simulink library "ddm"  (R2021b)
settings: Solver=VariableStepAuto  StartTime=0.0  StopTime=10.0  RelTol=1e-3
undefined symbols (not defined in the file or in its folder): ENUM_ADASACCSTA_ERROR, ENUM_ADASACCSTA_OFF, ENUM_ADASACCSTA_STANDBY, ENUM_ADASISASTA_OFF, ENUM_ALLOWMOV_ALLOWREADY, ENUM_APS, ENUM_BRKSTA_ERROR, ENUM_BRKSTA_OFF, ENUM_BRKSTA_ON, ENUM_CHGPREACTERRSTA_OBCPRE, ENUM_DCDCFAULTSTA_ANYFAULTLV1, ENUM_DCDCFAULTSTA_ANYFAULTLV2, ENUM_DRIVETRAIN_AWD, ENUM_DRIVETRAIN_FWD, ENUM_DRIVETRAIN_RWD, ENUM_DRSEATSTA_INVALID, ENUM_EDUDRTSTA_NORMAL, ENUM_EPBSTA_APPLIED, ENUM_EPBSTA_RELEASED, ENUM_HVBATTREADYPRE_READY, ENUM_MCUWARN_LV0, ENUM_MCUWARN_LV1, ENUM_MCUWARN_LV2, ENUM_MCUWARN_LV3, ENUM_MCUWARN_NOERROR, ENUM_OBCFAULTSTA_ANYFAULT, ENUM_PAS_R2F2, ENUM_PDFAULT_BATTPDFAIL, ENUM_PDFAULT_DCDCDISABLE, ENUM_PDFAULT_MCUDISABLE, ENUM_PDFAULT_MCUDISCHRG, ENUM_POWERSTA_OFF, ENUM_POWERSTA_ON, ENUM_POWERSTA_READY, ENUM_POWERSTA_STANDBY, ENUM_PRESSINDI_LOW, ENUM_PUFAULT_BATTUPFAIL, ENUM_PUFAULT_DCDCENABLEFAIL, ENUM_PUFAULT_PRECHRGCHKFAIL, ENUM_PUFAULT_SAFETYCHKFAIL, ENUM_PUSTATE_COMPLETED, ENUM_PWRSTASW_OFF, ENUM_PWRSTASW_OFFA, ENUM_PWRSTASW_OFFCHVCHRG, ENUM_PWRSTASW_OFFCLVCHRG, ENUM_PWRSTASW_ON, ENUM_PWRSTASW_ONHVCHRG, ENUM_PWRSTASW_READY, ENUM_PWRSTASW_STANDBY, ENUM_RANGESTA_12IN, ENUM_RANGESTA_12OUT, ENUM_SHIFTCOMMAND_D, ENUM_SHIFTCOMMAND_N, ENUM_SHIFTCOMMAND_P, ENUM_SHIFTCOMMAND_R, ENUM_ZONEMALFUNLV_1ST, ENUM_ZONEMALFUNLV_2ND, ENUM_ZONEMALFUNLV_3RD, ENUM_ZONEMALFUNLV_4TH, ENUM_ZONESPDCTRLMODE_ACC ... (+832)
libraries: hcu_lib x738, $bdroot x26, simulink x7
(part 10 of 25)

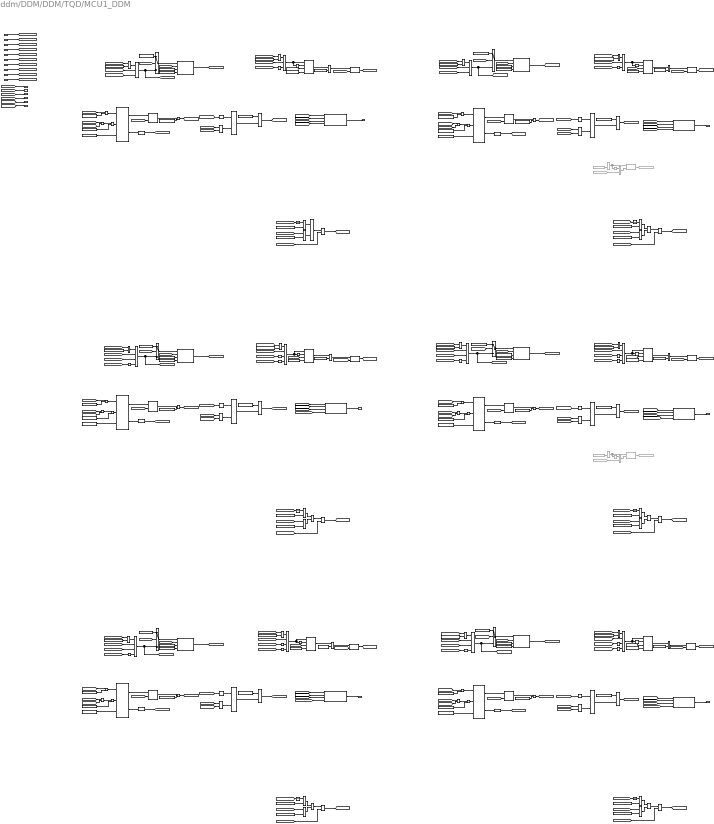
== system ddm/DDM/DDM/TQD/MCU1_DDM ==
  note: MCU_F1 Lost Comm (MCUF1NoCom)
  note: MCU_R1 Lost Comm (MCUR1NoCom)
  note: MCU_R1 Rolling Count Error (MCUR1RCErr)
  note: MCU_F1 Rolling Count Error (MCUF1RCErr)
  note: MCU_R1 Checksum Error (MCUR1CSErr)
  note: MCU_F1 Checksum Error (MCUF1CSErr)
  task_time_s : Inport
  VPMM_SysPwrSta_enum : Inport  Port=2
  No_CAN3_BUS_OFF : Inport  Port=3
  VDDM_MCUF1NoCom_flg : Inport  Port=4
  VDDM_MCUR1NoCom_flg : Inport  Port=5
  VDDM_MCUF1RCErr_flg : Inport  Port=6
  VDDM_MCUF1CSErr_flg : Inport  Port=7
  VDDM_MCUR1RCErr_flg : Inport  Port=8
  VDDM_MCUR1CSErr_flg : Inport  Port=9
  DTC_clear_request : Inport  Port=10
  Constant{1..2,9,24,35,46,53..54,62,66,79,86} (12 alike) : Constant  Value=ENUM_PWRSTASW_OFF
  Constant{3,10,25,40,55,75} (6 alike) : Constant  Value=ENUM_POWERSTA_OFF
  Constant{4,11,26,42,56,76} (6 alike) : Constant  Value=ENUM_POWERSTA_STANDBY
  Constant12 : Constant  Value=KDDM_MCUF1NoComDetSW_flg
  Constant13 : Constant  Value=KDDM_MCUF1NoComPassSW_flg
  Constant14 : Constant  Value=KDDM_MCUF1NoComDTC_cnt
  Constant15 : Constant  Value=KDDM_MCUF1NoComDFSSW_flg
  Constant16 : Constant  Value=KDDM_MCUR1NoComDTC_cnt
  Constant17 : Constant  Value=KDDM_MCUR1NoComPassTO_s
  Constant18 : Constant  Value=KDDM_MCUR1NoComPassTO_s
  Constant19 : Constant  Value=KDDM_MCUR1NoComDetTO_s
  Constant20 : Constant  Value=KDDM_MCUF1NoComCFSSW_flg
  Constant21 : Constant  Value=KDDM_MCUR1NoComCFSSW_flg
  Constant{22..23,38..39,73..74} (6 alike) : Constant  Value=FALSE
  Constant27 : Constant  Value=KDDM_MCUF1RCErrDetSW_flg
  Constant28 : Constant  Value=KDDM_MCUF1RCErrPassSW_flg
  Constant29 : Constant  Value=KDDM_MCUF1RCErrDTC_cnt
  Constant30 : Constant  Value=KDDM_MCUF1RCErrDFSSW_flg
  Constant31 : Constant  Value=KDDM_MCUR1RCErrDTC_cnt
  Constant32 : Constant  Value=KDDM_MCUR1RCErrPassTO_s
  Constant33 : Constant  Value=KDDM_MCUR1RCErrPassTO_s
  Constant34 : Constant  Value=KDDM_MCUR1RCErrDetTO_s
  Constant36 : Constant  Value=KDDM_MCUF1RCErrCFSSW_flg
  Constant37 : Constant  Value=KDDM_MCUR1RCErrCFSSW_flg
  Constant41 : Constant  Commented=on  Value=KDDM_MCUR1RCErrPassTO_s
  Constant43 : Constant  Commented=on  Value=KDDM_MCUR1RCErrPassTO_s
  Constant44 : Constant  Value=KDDM_MCUR1RCErrDetSW_flg
  Constant45 : Constant  Value=KDDM_MCUR1RCErrPassSW_flg
  Constant47 : Constant  Value=KDDM_MCUF1RCErrDTC_cnt
  Constant48 : Constant  Value=KDDM_MCUF1RCErrPassTO_s
  Constant49 : Constant  Value=KDDM_MCUR1RCErrDTC_cnt
  Constant5 : Constant  Value=KDDM_MCUR1NoComDetSW_flg
  Constant50 : Constant  Value=KDDM_MCUF1RCErrPassTO_s
  Constant51 : Constant  Value=KDDM_MCUF1RCErrDetTO_s
  Constant52 : Constant  Value=KDDM_MCUR1RCErrDFSSW_flg
  Constant57 : Constant  Value=KDDM_MCUF1CSErrDetSW_flg
  Constant58 : Constant  Value=KDDM_MCUF1CSErrPassSW_flg
  Constant59 : Constant  Value=KDDM_MCUF1CSErrDTC_cnt
  Constant6 : Constant  Value=KDDM_MCUR1NoComPassSW_flg
  Constant60 : Constant  Value=KDDM_MCUF1CSErrDFSSW_flg
  Constant61 : Constant  Value=KDDM_MCUR1CSErrDTC_cnt
  Constant63 : Constant  Value=KDDM_MCUR1CSErrPassTO_s
  Constant64 : Constant  Value=KDDM_MCUR1CSErrPassTO_s
  Constant65 : Constant  Value=KDDM_MCUR1CSErrDetTO_s
  Constant67 : Constant  Value=KDDM_MCUF1CSErrCFSSW_flg
  Constant68 : Constant  Value=KDDM_MCUF1NoComDTC_cnt
  Constant69 : Constant  Value=KDDM_MCUF1NoComPassTO_s
  Constant7 : Constant  Value=KDDM_MCUR1NoComDTC_cnt
  Constant70 : Constant  Value=KDDM_MCUF1NoComPassTO_s
  Constant71 : Constant  Value=KDDM_MCUF1NoComDetTO_s
  Constant72 : Constant  Value=KDDM_MCUR1CSErrCFSSW_flg
  Constant77 : Constant  Value=KDDM_MCUR1CSErrDetSW_flg
  Constant78 : Constant  Value=KDDM_MCUR1CSErrPassSW_flg
  Constant8 : Constant  Value=KDDM_MCUR1NoComDFSSW_flg
  Constant80 : Constant  Value=KDDM_MCUF1CSErrDTC_cnt
  Constant81 : Constant  Value=KDDM_MCUF1CSErrPassTO_s
  Constant82 : Constant  Value=KDDM_MCUR1CSErrDTC_cnt
  Constant83 : Constant  Value=KDDM_MCUF1CSErrPassTO_s
  Constant84 : Constant  Value=KDDM_MCUF1CSErrDetTO_s
  Constant85 : Constant  Value=KDDM_MCUR1CSErrDFSSW_flg
  DTC_Couter{1..6} (6 alike) : hcu_lib/Basic_Blocks/DTC_Couter
  DTC_Info{,1..5} (6 alike) : hcu_lib/Basic_Blocks/DTC_Info
  Data Type Conversion{1..6} (6 alike) : DataTypeConversion  OutDataTypeStr=uint8
  Equal{1..2,5,9..11,16,20..22,24,29} (12 alike) : RelationalOperator  Operator=~=  OutDataTypeStr=boolean  RndMeth=Simplest
  Equal12 : RelationalOperator  Commented=on  OutDataTypeStr=boolean  RndMeth=Simplest
  Equal{6,13,17,25,28,30} (6 alike) : RelationalOperator  OutDataTypeStr=boolean  RndMeth=Simplest
  Equal{3..4,7..8,14..15,18..19,26..27,31..32} (12 alike) : RelationalOperator  Operator===  OutDataTypeStr=boolean  RndMeth=Simplest
  Equal23 : RelationalOperator  Commented=on  OutDataTypeStr=boolean  RndMeth=Simplest
  From76 : From  Commented=on  GotoTag=VDDM_MCUR1RCErrRst_flg
  From94 : From  Commented=on  GotoTag=VDDM_MCUR1RCErrRst_flg
  Goto13 : Goto  Commented=on  GotoTag=VDDM_MCUR1RCErrPass_flg
  Goto14 : Goto  Commented=on  GotoTag=VDDM_MCUR1RCErrPass_flg
  Logical Operator{,1,4..7,10,16,18,25,27,36,38..42,49..50,55..57,60,63,69,71..75} (30 alike) : Logic  AllPortsSameDT=off  OutDataTypeStr=boolean
  Logical Operator{2,11,14,30} (4 alike) : Logic  Inputs=3  AllPortsSameDT=off  OutDataTypeStr=boolean
  Logical Operator{9,12,15,21,24,32,34,45..46,48,53,59,66,68,76..78,80} (18 alike) : Logic  Operator=OR  AllPortsSameDT=off  OutDataTypeStr=boolean
  Logical Operator{3,13,17,20,22,26,29,37,43,54,61,65,70,81..87} (20 alike) : Logic  Operator=NOT  AllPortsSameDT=off  OutDataTypeStr=boolean
  Logical Operator{19,23,28,31,51,58,64,67} (8 alike) : Logic  Inputs=4  AllPortsSameDT=off  OutDataTypeStr=boolean
  Logical Operator33 : Logic  Commented=on  Operator=NOT  AllPortsSameDT=off  OutDataTypeStr=boolean
  Logical Operator35 : Logic  Commented=on  Operator=NOT  AllPortsSameDT=off  OutDataTypeStr=boolean
  Logical Operator44 : Logic  Commented=on  Operator=OR  AllPortsSameDT=off  OutDataTypeStr=boolean
  Logical Operator62 : Logic  Commented=on  Operator=OR  AllPortsSameDT=off  OutDataTypeStr=boolean
  Relay{1..6} (6 alike) : Relay  OnSwitchValue=ONE_INT  OffSwitchValue=ZERO_INT
  SR_Latch{,1..4,6..9,11..19} (18 alike) : hcu_lib/Basic_Blocks/SR_Latch
  SR_Latch10 : hcu_lib/Basic_Blocks/SR_Latch  Commented=on
  SR_Latch5 : hcu_lib/Basic_Blocks/SR_Latch  Commented=on
  Switch{1..6} (6 alike) : Switch  Criteria=u2 ~= 0
  Test Detection Criteria{1..6} (6 alike) : hcu_lib/Basic_Blocks/Test Detection Criteria
  Timer{1..6} (6 alike) : hcu_lib/Basic_Blocks/Timer
  Unit Delay{,1..5} (6 alike) : UnitDelay  SampleTime=-1  HasFrameUpgradeWarning=on
  VDDM_MCUF1NoComDTC_raw32 : Outport
  VDDM_MCUR1NoComDTC_raw32 : Outport  Port=2
  VDDM_MCUF1RCErrDTC_raw32 : Outport  Port=3
  VDDM_MCUR1RCErrDTC_raw32 : Outport  Port=4
  VDDM_MCUF1CSErrDTC_raw32 : Outport  Port=5
  VDDM_MCUR1CSErrDTC_raw32 : Outport  Port=6
  VDDM_MCUF1NoComCFS_flg : Outport  Port=7
  VDDM_MCUF1RCErrCFS_flg : Outport  Port=8
  VDDM_MCUF1CSErrCFS_flg : Outport  Port=9
  VDDM_MCUR1NoComCFS_flg : Outport  Port=10
  VDDM_MCUR1RCErrCFS_flg : Outport  Port=11
  VDDM_MCUR1CSErrCFS_flg : Outport  Port=12
  wires:
  Constant12/1 -> Logical Operator5/2
  Equal3/1 -> Logical Operator4/1
  [VDDM_MCUF1NoCom_flg] -> Logical Operator30/3
  Constant10/1 -> Equal3/2
  Constant11/1 -> Equal4/2
  [DTC_clear_request] -> Logical Operator12/2
  Logical Operator12/1 -> [VDDM_MCUF1NoComCFSRls_flg]
  Equal21/1 -> Logical Operator30/1
  [VDDM_MCUF1NoComCFSRls_flg] -> SR_Latch/2
  Logical Operator5/1 -> DTC_Couter1/1
  Unit Delay/1 -> Equal3/1
  [No_CAN3_BUS_OFF] -> Logical Operator30/2
  Equal4/1 -> Logical Operator4/2
  [VPMM_SysPwrSta_enum] -> Unit Delay/1
  Timer1/1 -> Equal28/1
  DTC_Couter1/1 -> SR_Latch/1
  [VPMM_SysPwrSta_enum] -> Equal4/1
  [VDDM_MCUF1NoComDet_flg] -> Logical Operator5/1
  [VPMM_SysPwrSta_enum] -> Equal21/1
  Constant70/1 -> Timer1/4
  [task_time_s] -> Timer1/3
  Constant13/1 -> Logical Operator6/2
  Test Detection Criteria1/1 -> [VDDM_MCUF1NoComDet_flg]  "VDDM_MCUF1NoComDet_flg"
  Constant62/1 -> Equal21/2
  Logical Operator6/1 -> DTC_Couter1/2
  Logical Operator43/1 -> Timer1/2
  Constant69/1 -> Equal28/2
  Logical Operator4/1 -> Logical Operator12/1
  Logical Operator2/1 -> Logical Operator43/1, Timer1/1
  Equal1/1 -> Logical Operator2/1
  [VPMM_SysPwrSta_enum] -> Equal1/1
  [No_CAN3_BUS_OFF] -> Logical Operator2/2
  Constant1/1 -> Equal1/2
  [VDDM_MCUF1NoCom_flg] -> Logical Operator3/1
  Logical Operator3/1 -> Logical Operator2/3
  SR_Latch12/1 -> [VDDM_MCUF1NoComPass_flg]
  Logical Operator35/1 -> Logical Operator62/1
  Equal23/1 -> SR_Latch5/1, Logical Operator35/1
  From94/1 -> Logical Operator62/2
  Logical Operator62/1 -> SR_Latch5/2
  SR_Latch5/1 -> Goto14/1
  Constant41/1 -> Equal23/2
  [task_time_s] -> Test Detection Criteria1/2
  Constant68/1 -> Test Detection Criteria1/3
  Constant71/1 -> Test Detection Criteria1/4
  Equal28/1 -> SR_Latch12/1
  Constant14/1 -> DTC_Couter1/3
  [VDDM_MCUF1NoComPass_flg] -> Logical Operator34/1
  Logical Operator34/1 -> Logical Operator6/1
  [VDDM_MCUF1NoComCFSRls_flg] -> Logical Operator34/2
  Data Type Conversion2/1 -> [VDDM_MCUF1NoComDTC_cnt]  "VDDM_MCUF1NoComDTC_cnt"
  DTC_Couter1/2 -> Data Type Conversion2/1
  Constant15/1 -> Logical Operator55/1
  Logical Operator77/1 -> SR_Latch6/2
  Relay1/1 -> SR_Latch6/1
  Logical Operator55/1 -> [VDDM_MCUF1NoComDFS_flg]
  SR_Latch6/1 -> Logical Operator55/2
  [VDDM_MCUF1NoComDTC_cnt] -> Relay1/1
  [VDDM_MCUF1NoComDFSRls_flg] -> Logical Operator77/1
  [VDDM_MCUF1NoComCFS_flg] -> Logical Operator77/2
  Logical Operator66/1 -> SR_Latch13/2
  [VPMM_SysPwrSta_enum] -> Equal5/1
  [DTC_clear_request] -> Logical Operator9/2
  SR_Latch13/1 -> Logical Operator56/2
  Logical Operator17/1 -> Timer2/2
  [No_CAN3_BUS_OFF] -> Logical Operator11/2
  [VDDM_MCUR1NoComCFSRls_flg] -> SR_Latch1/2
  [VPMM_SysPwrSta_enum] -> Equal2/1
  Logical Operator16/1 -> Logical Operator9/1
  Equal5/1 -> Logical Operator14/1
  Relay2/1 -> SR_Latch13/1
  Constant19/1 -> Test Detection Criteria2/4
  Logical Operator57/1 -> DTC_Couter2/2
  Logical Operator11/1 -> Logical Operator17/1, Timer2/1
  Equal2/1 -> Logical Operator11/1
  [VDDM_MCUR1NoCom_flg] -> Logical Operator13/1
  Timer2/1 -> Equal6/1
  Equal7/1 -> Logical Operator16/1
  SR_Latch2/1 -> [VDDM_MCUR1NoComPass_flg]
  DTC_Couter2/2 -> Data Type Conversion1/1
  Constant3/1 -> Equal7/2
  [VDDM_MCUR1NoComDet_flg] -> Logical Operator18/1
  Constant5/1 -> Logical Operator18/2
  Test Detection Criteria2/1 -> [VDDM_MCUR1NoComDet_flg]  "VDDM_MCUR1NoComDet_flg"
  Logical Operator18/1 -> DTC_Couter2/1
  [VDDM_MCUR1NoComCFSRls_flg] -> Logical Operator15/2
  [VDDM_MCUR1NoComDFSRls_flg] -> Logical Operator66/1
  [VDDM_MCUR1NoComPass_flg] -> Logical Operator15/1
  [VDDM_MCUR1NoComDTC_cnt] -> Relay2/1
  Constant16/1 -> Test Detection Criteria2/3
  [VDDM_MCUR1NoComCFS_flg] -> Logical Operator66/2
  [VPMM_SysPwrSta_enum] -> Equal8/1
  Equal6/1 -> SR_Latch2/1
  [VDDM_MCUR1NoCom_flg] -> Logical Operator14/3
  Equal8/1 -> Logical Operator16/2
  Unit Delay1/1 -> Equal7/1
  Logical Operator15/1 -> Logical Operator57/1
  Constant2/1 -> Equal2/2
  Constant8/1 -> Logical Operator56/1
  Data Type Conversion1/1 -> [VDDM_MCUR1NoComDTC_cnt]  "VDDM_MCUR1NoComDTC_cnt"
  Logical Operator56/1 -> [VDDM_MCUR1NoComDFS_flg]
  Constant7/1 -> DTC_Couter2/3
  Constant4/1 -> Equal8/2
  Constant6/1 -> Logical Operator57/2
  Logical Operator9/1 -> [VDDM_MCUR1NoComCFSRls_flg]
  Constant18/1 -> Timer2/4
  Constant9/1 -> Equal5/2
  DTC_Couter2/1 -> SR_Latch1/1
  [No_CAN3_BUS_OFF] -> Logical Operator14/2
  [VPMM_SysPwrSta_enum] -> Unit Delay1/1
  Logical Operator13/1 -> Logical Operator11/3
  [task_time_s] -> Test Detection Criteria2/2
  Constant17/1 -> Equal6/2
  [task_time_s] -> Timer2/3
  [VDDM_MCUF1NoComCFS_flg] -> DTC_Info/3
  [VDDM_MCUF1NoComPass_flg] -> DTC_Info/2
  [VDDM_MCUF1NoComDet_flg] -> DTC_Info/1
  DTC_Info/1 -> VDDM_MCUF1NoComDTC_raw32/1  "VDDM_MCUF1NoComDTC_raw32"
  [VDDM_MCUR1NoComDet_flg] -> DTC_Info1/1
  DTC_Info1/1 -> VDDM_MCUR1NoComDTC_raw32/1  "VDDM_MCUR1NoComDTC_raw32"
  [VDDM_MCUR1NoComCFS_flg] -> DTC_Info1/3
  [VDDM_MCUR1NoComPass_flg] -> DTC_Info1/2
  task_time_s/1 -> [task_time_s]
  VPMM_SysPwrSta_enum/1 -> [VPMM_SysPwrSta_enum]
  No_CAN3_BUS_OFF/1 -> [No_CAN3_BUS_OFF]
  VDDM_MCUF1NoCom_flg/1 -> [VDDM_MCUF1NoCom_flg]
  DTC_clear_request/1 -> [DTC_clear_request]
  VDDM_MCUR1NoCom_flg/1 -> [VDDM_MCUR1NoCom_flg]
  SR_Latch/1 -> Logical Operator/1
  Logical Operator/1 -> [VDDM_MCUF1NoComCFS_flg]
  Constant20/1 -> Logical Operator/2
  Constant21/1 -> Logical Operator1/2
  SR_Latch1/1 -> Logical Operator1/1
  Logical Operator1/1 -> [VDDM_MCUR1NoComCFS_flg]
  [DTC_clear_request] -> DTC_Info/4
  [DTC_clear_request] -> DTC_Info1/4
  [DTC_clear_request] -> Switch6/2
  Switch6/1 -> Test Detection Criteria1/1
  Constant22/1 -> Switch6/1
  Logical Operator30/1 -> [VDDM_MCUF1NoComRst_flg], Switch6/3
  [DTC_clear_request] -> Switch1/2
  Switch1/1 -> Test Detection Criteria2/1
  Constant23/1 -> Switch1/1
  Equal14/1 -> Logical Operator36/1
  Unit Delay2/1 -> Equal14/1
  [VPMM_SysPwrSta_enum] -> Unit Delay2/1
  [VPMM_SysPwrSta_enum] -> Equal11/1
  Logical Operator42/1 -> DTC_Couter3/2
  Constant26/1 -> Equal15/2
  Equal13/1 -> SR_Latch7/1
  [VDDM_MCUR1RCErrCFSRls_flg] -> SR_Latch4/2
  [No_CAN3_BUS_OFF] -> Logical Operator31/2
  [VDDM_MCUF1RCErrCFSRls_flg] -> SR_Latch3/2
  Logical Operator37/1 -> Timer3/2
  [VDDM_MCUF1RCErrCFS_flg] -> Logical Operator46/2
  [DTC_clear_request] -> Logical Operator21/2
  [VPMM_SysPwrSta_enum] -> Equal15/1
  [VPMM_SysPwrSta_enum] -> Equal16/1
  Constant43/1 -> Equal12/2
  Timer3/1 -> Equal13/1
  Constant48/1 -> Equal13/2
  Logical Operator41/1 -> DTC_Couter4/2
  [VDDM_MCUR1RCErr_flg] -> Logical Operator22/1
  Equal15/1 -> Logical Operator36/2
  Logical Operator19/1 -> Timer4/1, Logical Operator26/1
  Test Detection Criteria3/1 -> [VDDM_MCUF1RCErrDet_flg]  "VDDM_MCUF1RCErrDet_flg"
  [VDDM_MCUF1RCErrCFSRls_flg] -> Logical Operator32/2
  Logical Operator44/1 -> SR_Latch10/2
  [VDDM_MCUF1RCErrDet_flg] -> Logical Operator38/1
  Constant51/1 -> Test Detection Criteria3/4
  [No_CAN3_BUS_OFF] -> Logical Operator28/2
  [VDDM_MCUR1RCErrDFSRls_flg] -> Logical Operator45/1
  Logical Operator32/1 -> Logical Operator42/1
  Constant30/1 -> Logical Operator39/1
  Equal11/1 -> Logical Operator31/1
  SR_Latch11/1 -> Logical Operator39/2
  [DTC_clear_request] -> Logical Operator48/2
  Logical Operator21/1 -> [VDDM_MCUF1RCErrCFSRls_flg]
  From76/1 -> Logical Operator44/2
  Data Type Conversion4/1 -> [VDDM_MCUF1RCErrDTC_cnt]  "VDDM_MCUF1RCErrDTC_cnt"
  Constant50/1 -> Timer3/4
  SR_Latch8/1 -> Logical Operator40/2
  [VPMM_SysPwrSta_enum] -> Equal9/1
  Constant34/1 -> Test Detection Criteria4/4
  [VDDM_MCUF1RCErr_flg] -> Logical Operator29/1
  [VDDM_MCUF1RCErrPass_flg] -> Logical Operator32/1
  [VDDM_MCUF1RCErrDFSRls_flg] -> Logical Operator46/1
  Constant46/1 -> Equal11/2
  Logical Operator46/1 -> SR_Latch11/2
  Constant29/1 -> DTC_Couter3/3
  Equal12/1 -> SR_Latch10/1, Logical Operator33/1
  SR_Latch9/1 -> [VDDM_MCUR1RCErrPass_flg]
  [VDDM_MCUF1RCErr_flg] -> Logical Operator31/3
  [VDDM_MCUR1RCErrCFSRls_flg] -> Logical Operator24/2
  [VPMM_SysPwrSta_enum] -> Equal10/1
  Relay4/1 -> SR_Latch8/1
  Equal10/1 -> Logical Operator19/1
  Logical Operator29/1 -> Logical Operator28/3
  Constant27/1 -> Logical Operator38/2
  Test Detection Criteria4/1 -> [VDDM_MCUR1RCErrDet_flg]  "VDDM_MCUR1RCErrDet_flg"
  [VDDM_MCUR1RCErrDet_flg] -> Logical Operator27/1
  Logical Operator36/1 -> Logical Operator21/1
  Relay3/1 -> SR_Latch11/1
  Constant25/1 -> Equal14/2
  SR_Latch10/1 -> Goto13/1
  Constant28/1 -> Logical Operator42/2
  DTC_Info2/1 -> VDDM_MCUF1RCErrDTC_raw32/1  "VDDM_MCUF1RCErrDTC_raw32"
  [VPMM_SysPwrSta_enum] -> Unit Delay3/1
  Constant35/1 -> Equal10/2
  DTC_Couter4/2 -> Data Type Conversion3/1
  Logical Operator33/1 -> Logical Operator44/1
  Constant42/1 -> Equal19/2
  [VDDM_MCUR1RCErrCFS_flg] -> Logical Operator45/2
  DTC_Couter4/1 -> SR_Latch4/1
  Constant40/1 -> Equal18/2
  DTC_Couter3/1 -> SR_Latch3/1
  Data Type Conversion3/1 -> [VDDM_MCUR1RCErrDTC_cnt]  "VDDM_MCUR1RCErrDTC_cnt"
  Constant52/1 -> Logical Operator40/1
  Logical Operator24/1 -> Logical Operator41/1
  Equal19/1 -> Logical Operator25/2
  [VDDM_MCUF1RCErrDet_flg] -> DTC_Info2/1
  Unit Delay3/1 -> Equal18/1
  [VDDM_MCUF1RCErrPass_flg] -> DTC_Info2/2
  DTC_Info3/1 -> VDDM_MCUR1RCErrDTC_raw32/1  "VDDM_MCUR1RCErrDTC_raw32"
  [task_time_s] -> Timer4/3
  [task_time_s] -> Test Detection Criteria3/2
  Constant24/1 -> Equal9/2
  [VDDM_MCUR1RCErrPass_flg] -> DTC_Info3/2
  Timer4/1 -> Equal17/1
  [VDDM_MCUR1RCErrPass_flg] -> Logical Operator24/1
  Logical Operator38/1 -> DTC_Couter3/1
  [VDDM_MCUR1RCErrDet_flg] -> DTC_Info3/1
  Logical Operator25/1 -> Logical Operator48/1
  Logical Operator27/1 -> DTC_Couter4/1
  Constant44/1 -> Logical Operator27/2
  [VDDM_MCUR1RCErr_flg] -> Logical Operator23/3
  Constant33/1 -> Timer4/4
  [No_CAN3_BUS_OFF] -> Logical Operator19/2
  Logical Operator40/1 -> [VDDM_MCUR1RCErrDFS_flg]
  [DTC_clear_request] -> Switch3/2
  Constant53/1 -> Equal16/2
  SR_Latch3/1 -> Logical Operator7/1
  [VDDM_MCUR1RCErrDTC_cnt] -> Relay4/1
  Logical Operator22/1 -> Logical Operator19/3
  Constant47/1 -> Test Detection Criteria3/3
  [task_time_s] -> Timer3/3
  Logical Operator39/1 -> [VDDM_MCUF1RCErrDFS_flg]
  Logical Operator7/1 -> [VDDM_MCUF1RCErrCFS_flg]
  SR_Latch7/1 -> [VDDM_MCUF1RCErrPass_flg]
  SR_Latch4/1 -> Logical Operator10/1
  Constant37/1 -> Logical Operator10/2
  Equal16/1 -> Logical Operator23/1
  [VDDM_MCUR1RCErrCFS_flg] -> DTC_Info3/3
  Logical Operator28/1 -> Timer3/1, Logical Operator37/1
  Constant32/1 -> Equal17/2
  [VDDM_MCUF1RCErrCFS_flg] -> DTC_Info2/3
  Constant45/1 -> Logical Operator41/2
  Logical Operator48/1 -> [VDDM_MCUR1RCErrCFSRls_flg]
  Constant38/1 -> Switch3/1
  Equal18/1 -> Logical Operator25/1
  [No_CAN3_BUS_OFF] -> Logical Operator23/2
  Equal17/1 -> SR_Latch9/1
  Constant49/1 -> DTC_Couter4/3
  Switch3/1 -> Test Detection Criteria3/1
  Logical Operator26/1 -> Timer4/2
  Constant31/1 -> Test Detection Criteria4/3
  Constant36/1 -> Logical Operator7/2
  [VPMM_SysPwrSta_enum] -> Equal19/1
  [DTC_clear_request] -> Switch2/2
  Logical Operator45/1 -> SR_Latch8/2
  [task_time_s] -> Test Detection Criteria4/2
  Switch2/1 -> Test Detection Criteria4/1
  Constant39/1 -> Switch2/1
  Logical Operator10/1 -> [VDDM_MCUR1RCErrCFS_flg]
  [DTC_clear_request] -> DTC_Info2/4
  [VDDM_MCUF1RCErrDTC_cnt] -> Relay3/1
  [DTC_clear_request] -> DTC_Info3/4
  DTC_Couter3/2 -> Data Type Conversion4/1
  Equal9/1 -> Logical Operator28/1
  Equal26/1 -> Logical Operator69/1
  Unit Delay4/1 -> Equal26/1
  [VPMM_SysPwrSta_enum] -> Unit Delay4/1
  [VPMM_SysPwrSta_enum] -> Equal24/1
  Logical Operator75/1 -> DTC_Couter5/2
  Constant56/1 -> Equal27/2
  Equal25/1 -> SR_Latch16/1
  [VDDM_MCUR1CSErrCFSRls_flg] -> SR_Latch15/2
  [No_CAN3_BUS_OFF] -> Logical Operator67/2
  [VDDM_MCUF1CSErrCFSRls_flg] -> SR_Latch14/2
  Logical Operator70/1 -> Timer5/2
  [VDDM_MCUF1CSErrCFS_flg] -> Logical Operator78/2
  [DTC_clear_request] -> Logical Operator53/2
  [VPMM_SysPwrSta_enum] -> Equal27/1
  [VPMM_SysPwrSta_enum] -> Equal29/1
  Timer5/1 -> Equal25/1
  Constant81/1 -> Equal25/2
  Logical Operator74/1 -> DTC_Couter6/2
  [VDDM_MCUR1CSErr_flg] -> Logical Operator54/1
  Equal27/1 -> Logical Operator69/2
  Logical Operator51/1 -> Timer6/1, Logical Operator61/1
  Test Detection Criteria5/1 -> [VDDM_MCUF1CSErrDet_flg]  "VDDM_MCUF1CSErrDet_flg"
  [VDDM_MCUF1CSErrCFSRls_flg] -> Logical Operator68/2
  [VDDM_MCUF1CSErrDet_flg] -> Logical Operator71/1
  Constant84/1 -> Test Detection Criteria5/4
  [No_CAN3_BUS_OFF] -> Logical Operator64/2
  [VDDM_MCUR1CSErrDFSRls_flg] -> Logical Operator76/1
  Logical Operator68/1 -> Logical Operator75/1
  Constant60/1 -> Logical Operator72/1
  Equal24/1 -> Logical Operator67/1
  SR_Latch19/1 -> Logical Operator72/2
  [DTC_clear_request] -> Logical Operator80/2
  Logical Operator53/1 -> [VDDM_MCUF1CSErrCFSRls_flg]
  Data Type Conversion6/1 -> [VDDM_MCUF1CSErrDTC_cnt]  "VDDM_MCUF1CSErrDTC_cnt"
  Constant83/1 -> Timer5/4
  SR_Latch17/1 -> Logical Operator73/2
  [VPMM_SysPwrSta_enum] -> Equal20/1
  Constant65/1 -> Test Detection Criteria6/4
  [VDDM_MCUF1CSErr_flg] -> Logical Operator65/1
  [VDDM_MCUF1CSErrPass_flg] -> Logical Operator68/1
  [VDDM_MCUF1CSErrDFSRls_flg] -> Logical Operator78/1
  Constant79/1 -> Equal24/2
  Logical Operator78/1 -> SR_Latch19/2
  Constant59/1 -> DTC_Couter5/3
  SR_Latch18/1 -> [VDDM_MCUR1CSErrPass_flg]
  [VDDM_MCUF1CSErr_flg] -> Logical Operator67/3
  [VDDM_MCUR1CSErrCFSRls_flg] -> Logical Operator59/2
  [VPMM_SysPwrSta_enum] -> Equal22/1
  Relay6/1 -> SR_Latch17/1
  Equal22/1 -> Logical Operator51/1
  Logical Operator65/1 -> Logical Operator64/3
  Constant57/1 -> Logical Operator71/2
  Test Detection Criteria6/1 -> [VDDM_MCUR1CSErrDet_flg]  "VDDM_MCUR1CSErrDet_flg"
  [VDDM_MCUR1CSErrDet_flg] -> Logical Operator63/1
  Logical Operator69/1 -> Logical Operator53/1
  Relay5/1 -> SR_Latch19/1
  Constant55/1 -> Equal26/2
  Constant58/1 -> Logical Operator75/2
  DTC_Info4/1 -> VDDM_MCUF1CSErrDTC_raw32/1  "VDDM_MCUF1CSErrDTC_raw32"
  [VPMM_SysPwrSta_enum] -> Unit Delay5/1
  Constant66/1 -> Equal22/2
  DTC_Couter6/2 -> Data Type Conversion5/1
  Constant76/1 -> Equal32/2
  [VDDM_MCUR1CSErrCFS_flg] -> Logical Operator76/2
  DTC_Couter6/1 -> SR_Latch15/1
  Constant75/1 -> Equal31/2
  DTC_Couter5/1 -> SR_Latch14/1
  Data Type Conversion5/1 -> [VDDM_MCUR1CSErrDTC_cnt]  "VDDM_MCUR1CSErrDTC_cnt"
  Constant85/1 -> Logical Operator73/1
  Logical Operator59/1 -> Logical Operator74/1
  Equal32/1 -> Logical Operator60/2
  [VDDM_MCUF1CSErrDet_flg] -> DTC_Info4/1
  Unit Delay5/1 -> Equal31/1
  [VDDM_MCUF1CSErrPass_flg] -> DTC_Info4/2
  DTC_Info5/1 -> VDDM_MCUR1CSErrDTC_raw32/1  "VDDM_MCUR1CSErrDTC_raw32"
  [task_time_s] -> Timer6/3
  [task_time_s] -> Test Detection Criteria5/2
  Constant54/1 -> Equal20/2
  [VDDM_MCUR1CSErrPass_flg] -> DTC_Info5/2
  Timer6/1 -> Equal30/1
  [VDDM_MCUR1CSErrPass_flg] -> Logical Operator59/1
  Logical Operator71/1 -> DTC_Couter5/1
  [VDDM_MCUR1CSErrDet_flg] -> DTC_Info5/1
  Logical Operator60/1 -> Logical Operator80/1
  Logical Operator63/1 -> DTC_Couter6/1
  Constant77/1 -> Logical Operator63/2
  [VDDM_MCUR1CSErr_flg] -> Logical Operator58/3
  Constant64/1 -> Timer6/4
  [No_CAN3_BUS_OFF] -> Logical Operator51/2
  Logical Operator73/1 -> [VDDM_MCUR1CSErrDFS_flg]
  [DTC_clear_request] -> Switch5/2
  Constant86/1 -> Equal29/2
  SR_Latch14/1 -> Logical Operator49/1
  [VDDM_MCUR1CSErrDTC_cnt] -> Relay6/1
  Logical Operator54/1 -> Logical Operator51/3
  Constant80/1 -> Test Detection Criteria5/3
  [task_time_s] -> Timer5/3
  Logical Operator72/1 -> [VDDM_MCUF1CSErrDFS_flg]
  Logical Operator49/1 -> [VDDM_MCUF1CSErrCFS_flg]
  SR_Latch16/1 -> [VDDM_MCUF1CSErrPass_flg]
  SR_Latch15/1 -> Logical Operator50/1
  Constant72/1 -> Logical Operator50/2
  Equal29/1 -> Logical Operator58/1
  [VDDM_MCUR1CSErrCFS_flg] -> DTC_Info5/3
  Logical Operator64/1 -> Timer5/1, Logical Operator70/1
  Constant63/1 -> Equal30/2
  [VDDM_MCUF1CSErrCFS_flg] -> DTC_Info4/3
  Constant78/1 -> Logical Operator74/2
  Logical Operator80/1 -> [VDDM_MCUR1CSErrCFSRls_flg]
  Constant73/1 -> Switch5/1
  Equal31/1 -> Logical Operator60/1
  [No_CAN3_BUS_OFF] -> Logical Operator58/2
  Equal30/1 -> SR_Latch18/1
  Constant82/1 -> DTC_Couter6/3
  Switch5/1 -> Test Detection Criteria5/1
  Logical Operator61/1 -> Timer6/2
  Constant61/1 -> Test Detection Criteria6/3
  Constant67/1 -> Logical Operator49/2
  [VPMM_SysPwrSta_enum] -> Equal32/1
  [DTC_clear_request] -> Switch4/2
  Logical Operator76/1 -> SR_Latch17/2
  [task_time_s] -> Test Detection Criteria6/2
  Switch4/1 -> Test Detection Criteria6/1
  Constant74/1 -> Switch4/1
  Logical Operator50/1 -> [VDDM_MCUR1CSErrCFS_flg]
  [DTC_clear_request] -> DTC_Info4/4
  [VDDM_MCUF1CSErrDTC_cnt] -> Relay5/1
  [DTC_clear_request] -> DTC_Info5/4
  DTC_Couter5/2 -> Data Type Conversion6/1
  Equal20/1 -> Logical Operator64/1
  [VDDM_MCUF1NoComCFS_flg] -> Logical Operator85/1
  [VDDM_MCUF1NoComCFS_flg] -> Logical Operator81/1
  Logical Operator81/1 -> Logical Operator31/4
  Logical Operator82/1 -> Logical Operator23/4
  [VDDM_MCUR1NoComCFS_flg] -> Logical Operator82/1
  Logical Operator83/1 -> Logical Operator67/4
  [VDDM_MCUF1NoComCFS_flg] -> Logical Operator83/1
  Logical Operator84/1 -> Logical Operator58/4
  [VDDM_MCUR1NoComCFS_flg] -> Logical Operator84/1
  VDDM_MCUF1RCErr_flg/1 -> [VDDM_MCUF1RCErr_flg]
  VDDM_MCUF1CSErr_flg/1 -> [VDDM_MCUF1CSErr_flg]
  VDDM_MCUR1RCErr_flg/1 -> [VDDM_MCUR1RCErr_flg]
  VDDM_MCUR1CSErr_flg/1 -> [VDDM_MCUR1CSErr_flg]
  Logical Operator85/1 -> Logical Operator28/4
  [VDDM_MCUF1NoComRst_flg] -> SR_Latch12/2
  [VDDM_MCUF1RCErrRst_flg] -> SR_Latch7/2
  Logical Operator31/1 -> [VDDM_MCUF1RCErrRst_flg], Switch3/3
  [VDDM_MCUR1NoComCFS_flg] -> Logical Operator20/1
  Logical Operator20/1 -> Logical Operator19/4
  Logical Operator86/1 -> Logical Operator51/4
  [VDDM_MCUR1NoComCFS_flg] -> Logical Operator86/1
  [VDDM_MCUF1NoComCFS_flg] -> Logical Operator87/1
  Logical Operator87/1 -> Logical Operator64/4
  Logical Operator67/1 -> [VDDM_MCUF1CSErrRst_flg], Switch5/3
  [VDDM_MCUF1CSErrRst_flg] -> SR_Latch16/2
  Logical Operator14/1 -> [VDDM_MCUR1NoComRst_flg], Switch1/3
  [VDDM_MCUR1NoComRst_flg] -> SR_Latch2/2
  Logical Operator23/1 -> [VDDM_MCUR1RCErrRst_flg], Switch2/3
  [VDDM_MCUR1RCErrRst_flg] -> SR_Latch9/2
  Logical Operator58/1 -> [VDDM_MCUR1CSErrRst_flg], Switch4/3
  [VDDM_MCUR1CSErrRst_flg] -> SR_Latch18/2
  [VDDM_MCUF1NoComCFS_flg] -> VDDM_MCUF1NoComCFS_flg/1
  [VDDM_MCUF1CSErrCFS_flg] -> VDDM_MCUF1CSErrCFS_flg/1
  [VDDM_MCUR1CSErrCFS_flg] -> VDDM_MCUR1CSErrCFS_flg/1
  [VDDM_MCUR1RCErrCFS_flg] -> VDDM_MCUR1RCErrCFS_flg/1
  [VDDM_MCUR1NoComCFS_flg] -> VDDM_MCUR1NoComCFS_flg/1
  [VDDM_MCUF1RCErrCFS_flg] -> VDDM_MCUF1RCErrCFS_flg/1

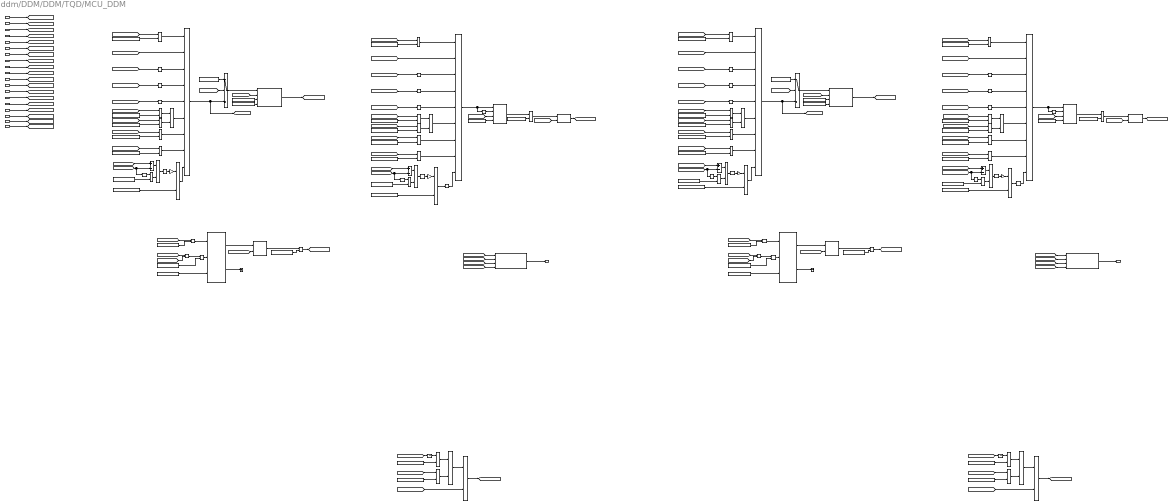
== system ddm/DDM/DDM/TQD/MCU_DDM ==
  note: Front Motor Torque Response Error (FrMCUTqErr)
  note: Fail Safe During Detection
  note: Test Pass Creteria
  note: Test Dtection Criteria
  note: Fail Safe After Detection
  note: Fail Safe During Detection
  note: Test Pass Creteria
  note: Rear Motor Torque Response Error (RrMCUTqErr)
  note: Test Dtection Criteria
  note: Fail Safe After Detection
  task_time_s : Inport
  VPMM_SysPwrSta_enum : Inport  Port=2
  No_CAN3_BUS_OFF : Inport  Port=3
  VDDM_MCUF1NoComCFS_flg : Inport  Port=4
  VDDM_MCUF1RCErrCFS_flg : Inport  Port=5
  VDDM_MCUF1CSErrCFS_flg : Inport  Port=6
  VINP_VehSpeed_kph : Inport  Port=7
  VINP_FrEDUDrtSta_flg : Inport  Port=8
  VINP_FrEDURealTMTq_Nm : Inport  Port=9
  VTQR_FrTMTqReq_Nm : Inport  Port=10
  VDDM_MCUR1NoComCFS_flg : Inport  Port=11
  VDDM_MCUR1RCErrCFS_flg : Inport  Port=12
  VDDM_MCUR1CSErrCFS_flg : Inport  Port=13
  VINP_RrEDUDrtSta_flg : Inport  Port=14
  VINP_RrEDURealTMTq_Nm : Inport  Port=15
  VTQR_RrTMTqReq_Nm : Inport  Port=16
  VINP_MCUWarnF_enum : Inport  Port=17
  VINP_MCUWarnR_enum : Inport  Port=18
  DTC_clear_request : Inport  Port=19
  Abs{,1..7} (8 alike) : Abs
  Add{,1..3} (4 alike) : Sum  Inputs=+-
  Constant{,1,47..48} (4 alike) : Constant  Value=eps
  Constant10 : Constant  Value=ENUM_POWERSTA_OFF
  Constant11 : Constant  Value=ENUM_POWERSTA_STANDBY
  Constant12 : Constant  Value=KDDM_RrMCUTqErrDetSW_flg
  Constant13 : Constant  Value=KDDM_FrMCUTqErrDetSW_flg
  Constant14 : Constant  Value=KDDM_FrMCUTqErrPassSW_flg
  Constant15 : Constant  Value=KDDM_FrMCUTqErrDet_pct
  Constant{4,16,26,32} (4 alike) : Constant  Value=ENUM_MCUWARN_LV0
  Constant{17,27,33,44} (4 alike) : Constant  Value=ENUM_PWRSTASW_OFF
  Constant18 : Constant  Value=ENUM_POWERSTA_OFF
  Constant19 : Constant  Value=ENUM_POWERSTA_STANDBY
  Constant2 : Constant  Value=KDDM_FrMCUTqErrCFSSW_flg
  Constant{5,20,29,34} (4 alike) : Constant  Value=ENUM_MCUWARN_NOERROR
  Constant{6,21,30,35} (4 alike) : Constant  Value=ENUM_EDUDRTSTA_NORMAL
  Constant22 : Constant  Value=KDDM_RrMCUTqErrPassSW_flg
  Constant23 : Constant  Value=KDDM_RrMCUTqErrCFSSW_flg
  Constant24 : Constant  Value=FALSE
  Constant25 : Constant  Value=KDDM_RrMCUTqErrDet_pct
  Constant28 : Constant  Value=KDDM_RrMCUTqErrDTC_cnt
  Constant3 : Constant  Value=KDDM_FrMCUTqErrDet_kph
  Constant31 : Constant  Value=KDDM_RrMCUTqErrDet_kph
  Constant36 : Constant  Value=KDDM_RrMCUTqErrPassTO_s
  Constant37 : Constant  Value=KDDM_RrMCUTqErrDetTO_s
  Constant38 : Constant  Value=KDDM_RrMCUTqErrDet_kph
  Constant39 : Constant  Value=KDDM_RrMCUTqErrPassTO_s
  Constant40 : Constant  Value=KDDM_RrMCUTqErrDTC_cnt
  Constant41 : Constant  Value=KDDM_FrMCUTqErrDet_pct
  Constant42 : Constant  Value=FALSE
  Constant43 : Constant  Value=KDDM_FrMCUTqErrDTC_cnt
  Constant45 : Constant  Value=KDDM_FrMCUTqErrPassTO_s
  Constant46 : Constant  Value=KDDM_FrMCUTqErrDetTO_s
  Constant7 : Constant  Value=KDDM_FrMCUTqErrDet_kph
  Constant70 : Constant  Value=KDDM_FrMCUTqErrPassTO_s
  Constant8 : Constant  Value=KDDM_FrMCUTqErrDTC_cnt
  Constant9 : Constant  Value=KDDM_RrMCUTqErrDet_pct
  DTC_Couter1 : hcu_lib/Basic_Blocks/DTC_Couter
  DTC_Couter2 : hcu_lib/Basic_Blocks/DTC_Couter
  DTC_Info : hcu_lib/Basic_Blocks/DTC_Info
  DTC_Info1 : hcu_lib/Basic_Blocks/DTC_Info
  Divide{,1..3} (4 alike) : Product  Inputs=*/
  Equal{1,3..4,6..10,15..16,21..22,30..31,33..34} (16 alike) : RelationalOperator  Operator===  OutDataTypeStr=boolean  RndMeth=Simplest
  Equal{5,11..12,17..18,27} (6 alike) : RelationalOperator  OutDataTypeStr=boolean  RndMeth=Simplest
  Equal{2,13,19,23} (4 alike) : RelationalOperator  Operator=>  OutDataTypeStr=boolean  RndMeth=Simplest
  Equal{14,20,24,26} (4 alike) : RelationalOperator  Operator=~=  OutDataTypeStr=boolean  RndMeth=Simplest
  Gain{,1..3} (4 alike) : Gain  Gain=100  OutDataTypeStr=single
  Logical Operator{1..2,5,12,16,20,25,31} (8 alike) : Logic  Operator=OR  AllPortsSameDT=off  OutDataTypeStr=boolean
  Logical Operator{3,7,9..10,13..15,17,21..23,26,28,34..35,37} (16 alike) : Logic  Operator=NOT  AllPortsSameDT=off  OutDataTypeStr=boolean
  Logical Operator{11,18,27,30} (4 alike) : Logic  Inputs=9  AllPortsSameDT=off  OutDataTypeStr=boolean
  Logical Operator{4,6,8,19,24,29,32..33} (8 alike) : Logic  AllPortsSameDT=off  OutDataTypeStr=boolean
  Max{,1..3} (4 alike) : MinMax  Function=max  Inputs=2
  SR_Latch{1..3,12} (4 alike) : hcu_lib/Basic_Blocks/SR_Latch
  Switch1 : Switch  Criteria=u2 ~= 0
  Switch6 : Switch  Criteria=u2 ~= 0
  Terminator : Terminator
  Terminator1 : Terminator
  Test Detection Criteria1 : hcu_lib/Basic_Blocks/Test Detection Criteria
  Test Detection Criteria2 : hcu_lib/Basic_Blocks/Test Detection Criteria
  Timer1 : hcu_lib/Basic_Blocks/Timer
  Timer2 : hcu_lib/Basic_Blocks/Timer
  Unit Delay : UnitDelay  SampleTime=-1  HasFrameUpgradeWarning=on
  Unit Delay1 : UnitDelay  SampleTime=-1  HasFrameUpgradeWarning=on
  VDDM_FrMCUTqErrDTC_raw32 : Outport
  VDDM_RrMCUTqErrDTC_raw32 : Outport  Port=2
  wires:
  Equal26/1 -> Logical Operator30/1
  Constant44/1 -> Equal26/2
  [VPMM_SysPwrSta_enum] -> Equal26/1
  Logical Operator12/1 -> [VDDM_FrMCUTqErrCFSRls_flg]
  Constant11/1 -> Equal4/2
  [VPMM_SysPwrSta_enum] -> Unit Delay/1
  [DTC_clear_request] -> Logical Operator12/2
  Equal3/1 -> Logical Operator4/1
  [VPMM_SysPwrSta_enum] -> Equal4/1
  [No_CAN_BUS_OFF] -> Logical Operator30/2
  Equal4/1 -> Logical Operator4/2
  Unit Delay/1 -> Equal3/1
  Logical Operator4/1 -> Logical Operator12/1
  Constant10/1 -> Equal3/2
  Constant3/1 -> Equal2/2
  [VINP_VehSpeed_kph] -> Equal2/1
  Constant4/1 -> Equal6/2
  Constant5/1 -> Equal7/2
  Equal6/1 -> Logical Operator1/1
  Equal7/1 -> Logical Operator1/2
  Logical Operator1/1 -> Logical Operator30/6
  [VINP_FrEDUDrtSta_flg] -> Equal10/1
  Constant6/1 -> Equal10/2
  Equal10/1 -> Logical Operator30/7
  Equal2/1 -> Logical Operator30/8
  [VDDM_MCUF1CSErrCFS_flg] -> Logical Operator10/1
  [VDDM_MCUF1RCErrCFS_flg] -> Logical Operator9/1
  Logical Operator9/1 -> Logical Operator30/4
  [VDDM_MCUF1NoComCFS_flg] -> Logical Operator7/1
  Logical Operator7/1 -> Logical Operator30/3
  Logical Operator10/1 -> Logical Operator30/5
  Add/1 -> Divide/1
  Abs/1 -> Gain/1
  Divide/1 -> Abs/1
  [VINP_FrEDURealTMTq_Nm] -> Add/1
  [VTQR_FrTMTqReq_Nm] -> Abs4/1, Add/2
  Gain/1 -> Equal12/1
  Equal12/1 -> Logical Operator30/9
  Constant15/1 -> Equal12/2
  Logical Operator2/1 -> Logical Operator11/6
  [VINP_FrEDUDrtSta_flg] -> Equal1/1
  Constant20/1 -> Equal16/2
  [VDDM_MCUF1NoComCFS_flg] -> Logical Operator13/1
  Equal1/1 -> Logical Operator11/7
  Constant16/1 -> Equal15/2
  Equal13/1 -> Logical Operator11/8
  Logical Operator14/1 -> Logical Operator11/4
  [VDDM_MCUF1RCErrCFS_flg] -> Logical Operator14/1
  Constant7/1 -> Equal13/2
  Constant21/1 -> Equal1/2
  [VINP_VehSpeed_kph] -> Equal13/1
  Logical Operator3/1 -> Logical Operator11/5
  [VDDM_MCUF1CSErrCFS_flg] -> Logical Operator3/1
  Constant17/1 -> Equal14/2
  [No_CAN_BUS_OFF] -> Logical Operator11/2
  Equal16/1 -> Logical Operator2/2
  [VPMM_SysPwrSta_enum] -> Equal14/1
  Equal14/1 -> Logical Operator11/1
  Equal15/1 -> Logical Operator2/1
  Logical Operator13/1 -> Logical Operator11/3
  Equal11/1 -> Logical Operator15/1
  Logical Operator15/1 -> Logical Operator11/9
  [VDDM_MCUR1CSErrCFS_flg] -> Logical Operator17/1
  Equal8/1 -> Logical Operator18/7
  Logical Operator22/1 -> Logical Operator18/4
  [VDDM_MCUR1RCErrCFS_flg] -> Logical Operator22/1
  Equal33/1 -> Logical Operator16/1
  [VINP_MCUWarnR_enum] -> Equal33/1
  [VINP_VehSpeed_kph] -> Equal23/1
  Constant38/1 -> Equal19/2
  [VDDM_MCUR1CSErrCFS_flg] -> Logical Operator26/1
  Constant27/1 -> Equal20/2
  Logical Operator21/1 -> Logical Operator18/3
  Equal21/1 -> Logical Operator25/1
  Logical Operator26/1 -> Logical Operator18/5
  [VINP_VehSpeed_kph] -> Equal19/1
  Constant18/1 -> Equal30/2
  [VPMM_SysPwrSta_enum] -> Equal20/1
  [No_CAN_BUS_OFF] -> Logical Operator18/2
  Logical Operator23/1 -> Logical Operator18/9
  Logical Operator29/1 -> Logical Operator20/1
  Equal20/1 -> Logical Operator18/1
  [VINP_MCUWarnR_enum] -> Equal34/1
  Logical Operator17/1 -> Logical Operator27/5
  Equal34/1 -> Logical Operator16/2
  Equal31/1 -> Logical Operator29/2
  [VPMM_SysPwrSta_enum] -> Equal31/1
  Equal18/1 -> Logical Operator27/9
  [VDDM_MCUR1NoComCFS_flg] -> Logical Operator35/1
  Equal22/1 -> Logical Operator25/2
  Constant33/1 -> Equal24/2
  Equal23/1 -> Logical Operator27/8
  [VINP_RrEDURealTMTq_Nm] -> Add2/1
  Constant26/1 -> Equal21/2
  Equal19/1 -> Logical Operator18/8
  Equal9/1 -> Logical Operator27/7
  Unit Delay1/1 -> Equal30/1
  [VDDM_MCUR1RCErrCFS_flg] -> Logical Operator37/1
  Constant30/1 -> Equal8/2
  Constant29/1 -> Equal22/2
  [VDDM_MCUR1NoComCFS_flg] -> Logical Operator21/1
  Constant35/1 -> Equal9/2
  Logical Operator35/1 -> Logical Operator27/3
  Constant32/1 -> Equal33/2
  [VINP_RrEDUDrtSta_flg] -> Equal9/1
  Constant34/1 -> Equal34/2
  [No_CAN_BUS_OFF] -> Logical Operator27/2
  [VPMM_SysPwrSta_enum] -> Unit Delay1/1
  Equal30/1 -> Logical Operator29/1
  Constant31/1 -> Equal23/2
  Logical Operator25/1 -> Logical Operator18/6
  Constant19/1 -> Equal31/2
  [DTC_clear_request] -> Logical Operator20/2
  Logical Operator16/1 -> Logical Operator27/6
  Equal24/1 -> Logical Operator27/1
  [VPMM_SysPwrSta_enum] -> Equal24/1
  [VINP_RrEDUDrtSta_flg] -> Equal8/1
  Logical Operator37/1 -> Logical Operator27/4
  Logical Operator20/1 -> [VDDM_RrMCUTqErrCFSRls_flg]
  Logical Operator11/1 -> Logical Operator34/1, Timer1/1
  [task_time_s] -> Test Detection Criteria1/2
  [task_time_s] -> Timer1/3
  Constant42/1 -> Switch6/1
  Test Detection Criteria1/1 -> [VDDM_FrMCUTqErrDet_flg]  "VDDM_FrMCUTqErrDet_flg"
  Equal27/1 -> SR_Latch12/1
  Logical Operator34/1 -> Timer1/2
  Timer1/1 -> Equal27/1
  Constant43/1 -> Test Detection Criteria1/3
  Switch6/1 -> Test Detection Criteria1/1
  SR_Latch12/1 -> [VDDM_FrMCUTqErrPass_flg]
  Logical Operator30/1 -> [VDDM_FrMCUTqErrRst_flg], Switch6/3
  Constant46/1 -> Test Detection Criteria1/4
  Constant70/1 -> Timer1/4
  Constant45/1 -> Equal27/2
  [VDDM_FrMCUTqErrRst_flg] -> SR_Latch12/2
  [DTC_clear_request] -> Switch6/2
  [VDDM_FrMCUTqErrDet_flg] -> DTC_Info/1
  Logical Operator19/1 -> [VDDM_FrMCUTqErrCFS_flg]
  [VDDM_FrMCUTqErrCFSRls_flg] -> SR_Latch1/2
  DTC_Info/1 -> VDDM_FrMCUTqErrDTC_raw32/1  "VDDM_FrMCUTqErrDTC_raw32"
  [VDDM_FrMCUTqErrCFSRls_flg] -> Logical Operator5/2
  DTC_Couter1/1 -> SR_Latch1/1
  [VDDM_FrMCUTqErrPass_flg] -> Logical Operator5/1
  Constant13/1 -> Logical Operator6/2
  Logical Operator5/1 -> Logical Operator8/1
  [DTC_clear_request] -> DTC_Info/4
  Logical Operator6/1 -> DTC_Couter1/1
  Logical Operator8/1 -> DTC_Couter1/2
  SR_Latch1/1 -> Logical Operator19/1
  [VDDM_FrMCUTqErrDet_flg] -> Logical Operator6/1
  Constant2/1 -> Logical Operator19/2
  Constant14/1 -> Logical Operator8/2
  [VDDM_FrMCUTqErrCFS_flg] -> DTC_Info/3
  Constant8/1 -> DTC_Couter1/3
  [VDDM_FrMCUTqErrPass_flg] -> DTC_Info/2
  DTC_Couter1/2 -> Terminator/1
  DTC_Couter2/1 -> SR_Latch2/1
  [DTC_clear_request] -> Switch1/2
  [VDDM_RrMCUTqErrCFSRls_flg] -> Logical Operator31/2
  [VDDM_RrMCUTqErrCFSRls_flg] -> SR_Latch2/2
  Test Detection Criteria2/1 -> [VDDM_RrMCUTqErrDet_flg]  "VDDM_RrMCUTqErrDet_flg"
  [VDDM_RrMCUTqErrDet_flg] -> DTC_Info1/1
  Constant12/1 -> Logical Operator32/2
  DTC_Info1/1 -> VDDM_RrMCUTqErrDTC_raw32/1  "VDDM_RrMCUTqErrDTC_raw32"
  [DTC_clear_request] -> DTC_Info1/4
  SR_Latch3/1 -> [VDDM_RrMCUTqErrPass_flg]
  Logical Operator24/1 -> [VDDM_RrMCUTqErrCFS_flg]
  Constant22/1 -> Logical Operator33/2
  Constant23/1 -> Logical Operator24/2
  [VDDM_RrMCUTqErrCFS_flg] -> DTC_Info1/3
  SR_Latch2/1 -> Logical Operator24/1
  Constant39/1 -> Timer2/4
  Logical Operator32/1 -> DTC_Couter2/1
  Logical Operator33/1 -> DTC_Couter2/2
  [VDDM_RrMCUTqErrPass_flg] -> Logical Operator31/1
  DTC_Couter2/2 -> Terminator1/1
  Logical Operator31/1 -> Logical Operator33/1
  Constant24/1 -> Switch1/1
  [task_time_s] -> Timer2/3
  Timer2/1 -> Equal5/1
  Constant40/1 -> DTC_Couter2/3
  [VDDM_RrMCUTqErrPass_flg] -> DTC_Info1/2
  [task_time_s] -> Test Detection Criteria2/2
  Equal5/1 -> SR_Latch3/1
  Constant28/1 -> Test Detection Criteria2/3
  Logical Operator27/1 -> [VDDM_RrMCUTqErrRst_flg], Switch1/3
  Constant37/1 -> Test Detection Criteria2/4
  [VDDM_RrMCUTqErrRst_flg] -> SR_Latch3/2
  Switch1/1 -> Test Detection Criteria2/1
  [VDDM_RrMCUTqErrDet_flg] -> Logical Operator32/1
  Logical Operator28/1 -> Timer2/2
  Constant36/1 -> Equal5/2
  Logical Operator18/1 -> Logical Operator28/1, Timer2/1
  task_time_s/1 -> [task_time_s]
  VPMM_SysPwrSta_enum/1 -> [VPMM_SysPwrSta_enum]
  No_CAN3_BUS_OFF/1 -> [No_CAN_BUS_OFF]
  VDDM_MCUF1NoComCFS_flg/1 -> [VDDM_MCUF1NoComCFS_flg]
  VDDM_MCUF1RCErrCFS_flg/1 -> [VDDM_MCUF1RCErrCFS_flg]
  VDDM_MCUF1CSErrCFS_flg/1 -> [VDDM_MCUF1CSErrCFS_flg]
  VINP_FrEDUDrtSta_flg/1 -> [VINP_FrEDUDrtSta_flg]
  VINP_VehSpeed_kph/1 -> [VINP_VehSpeed_kph]
  VINP_FrEDURealTMTq_Nm/1 -> [VINP_FrEDURealTMTq_Nm]
  VTQR_FrTMTqReq_Nm/1 -> [VTQR_FrTMTqReq_Nm]
  VDDM_MCUR1NoComCFS_flg/1 -> [VDDM_MCUR1NoComCFS_flg]
  VDDM_MCUR1RCErrCFS_flg/1 -> [VDDM_MCUR1RCErrCFS_flg]
  VDDM_MCUR1CSErrCFS_flg/1 -> [VDDM_MCUR1CSErrCFS_flg]
  VINP_RrEDUDrtSta_flg/1 -> [VINP_RrEDUDrtSta_flg]
  VINP_RrEDURealTMTq_Nm/1 -> [VINP_RrEDURealTMTq_Nm]
  VTQR_RrTMTqReq_Nm/1 -> [VTQR_RrTMTqReq_Nm]
  DTC_clear_request/1 -> [DTC_clear_request]
  VINP_MCUWarnF_enum/1 -> [VINP_MCUWarnF_enum]
  VINP_MCUWarnR_enum/1 -> [VINP_MCUWarnR_enum]
  [VINP_MCUWarnF_enum] -> Equal6/1
  [VINP_MCUWarnF_enum] -> Equal7/1
  [VINP_MCUWarnF_enum] -> Equal15/1
  [VINP_MCUWarnF_enum] -> Equal16/1
  [VINP_MCUWarnR_enum] -> Equal21/1
  [VINP_MCUWarnR_enum] -> Equal22/1
  Constant/1 -> Max/2
  Abs4/1 -> Max/1
  Max/1 -> Divide/2
  Max1/1 -> Divide1/2
  Constant1/1 -> Max1/2
  Abs1/1 -> Gain1/1
  Gain1/1 -> Equal11/1
  Add1/1 -> Divide1/1
  Constant41/1 -> Equal11/2
  Abs5/1 -> Max1/1
  Divide1/1 -> Abs1/1
  [VINP_FrEDURealTMTq_Nm] -> Add1/1
  [VTQR_FrTMTqReq_Nm] -> Abs5/1, Add1/2
  Abs6/1 -> Max2/1
  [VTQR_RrTMTqReq_Nm] -> Add2/2, Abs6/1
  Abs2/1 -> Gain2/1
  Max2/1 -> Divide2/2
  Constant47/1 -> Max2/2
  Constant25/1 -> Equal18/2
  Divide2/1 -> Abs2/1
  Add2/1 -> Divide2/1
  Gain2/1 -> Equal18/1
  Gain3/1 -> Equal17/1
  [VTQR_RrTMTqReq_Nm] -> Add3/2, Abs7/1
  [VINP_RrEDURealTMTq_Nm] -> Add3/1
  Max3/1 -> Divide3/2
  Abs7/1 -> Max3/1
  Divide3/1 -> Abs3/1
  Constant48/1 -> Max3/2
  Constant9/1 -> Equal17/2
  Add3/1 -> Divide3/1
  Abs3/1 -> Gain3/1
  Equal17/1 -> Logical Operator23/1
